simulink model "DEMOSYSTEM"  (R2015b)
settings: Solver=ode3  StartTime=0.0  StopTime=inf  FixedStep=T  RelTol=1e-3
InitFcn:
  | clear variables
  | T = 0.005; %Sampling time
  | 
  | % Impact detect subsys
  | %footExtensionRange = 17;        % 17[deg] hip angle at which foot extends/retracts
  | impactGeometryCondition = 10;   % 10 [deg] angle for geometric condition to check for impacts
  | impactGeometryConditionTol = 1; % 1 [deg] tolerance for impactGeometryCondition
  | 
  | impactCondi1 = 9*pi/180; % 9 [rad] retract
  | impactCondi2 = 1*pi/180; % 1 [rad] extend
  | 
  | % VC subsys
  | st_range = pi/18;
  | theta_retract = st_range;
  | theta_extend = -1*pi/180;
  | 
  | %refGenCoeffs = [ -1.0000, -0.9000, -1.0000, -1.2000, 1.9000, 2.4000, 1.3000, 1.1000, 1.0000];% MSC
  | refGenCoeffs = [ -1.0000, -0.9659, -0.8000, -0.8000, 1.3000, 1.4000, 1.3000, 1.2000, 1.0000];% Justin - slow
  | 
  | % PID subsys
  | feedbackP = 0.3;
  | feedbackD = 0.092;
  | 
  | % Observer gains
  | L1 = 200;
  | L2 = 10000;
  | A = [ 0 1 ;  0 0 ];
  | C = [ 1 0 ];
StopFcn:
  | % save file to results folder if it ran for longer than 10 seconds
  | 
  | %if(controlData.ref.Time(end) > 10)
  | %  name = datestr(now);
  | %  name = strrep(name,' ','_');
  | %  name = strrep(name,':','-');
  | %  name = strcat('results/',name);
  | %  save(name)
  | %end
  | 
  | %% display demo mode params:
  | disp('=====DEMO MODE=====');
undefined symbols (not defined in the file or in its folder): National_Instruments, PCI
libraries: simulink x8, sldrtlib x6, simulink_extras x1
settings Model: Creator=mounir  LastModifiedBy=mounir
settings DataIOCC: SaveFormat=Array
settings HardwareCC: ProdBitPerPointer=32  ProdLargestAtomicFloat=None  ProdIntDivRoundTo=Undefined  ProdEndianess=Unspecified  ProdWordSize=32  ProdHWDeviceType=32-bit Generic
settings GRTTargetCC: GeneratePreprocessorConditionals=Disable all
settings ConfigComp: CovModelRefEnable=Off

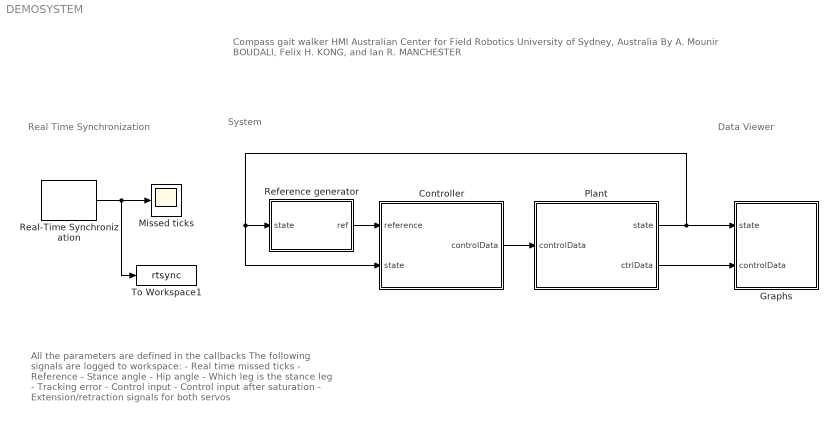
== system DEMOSYSTEM ==
  note: Compass gait walker HMI
      | Australian Center for Field Robotics
      | University of Sydney, Australia
      | By A. Mounir BOUDALI, Felix H. KONG, and Ian R. MANCHESTER
  note: All the parameters are defined in the callbacks
      |
      | The following signals are logged to workspace:
      | - Real time missed ticks
      | - Reference
      | - Stance angle
      | - Hip angle
      | - Which leg is the stance leg
      | - Tracking error
      | - Control input
      | - Control input after saturation
      | - Extension/retraction signals for both servos
  note: System
  note: Data Viewer
  note: Real Time Synchronization
  Controller : Subsystem
  Graphs : Subsystem
  Missed ticks : Scope
  Plant : Subsystem
  Real-Time Synchronization : sldrtlib/Real-Time Synchronization  SampleTime=T  MaxMissedTicks=100  ShowMissedTicks=on  YieldWhenWaiting=on
  Reference generator : Subsystem
  To Workspace1 : ToWorkspace  VariableName=rtsync  SaveFormat=Timeseries  SampleTime=T
  wires:
  Plant/1(state) -> Graphs/1(state), Reference generator/1(state), Controller/2(state)
  Controller/1(controlData) -> Plant/1(controlData)
  Reference generator/1(ref) -> Controller/1(reference)
  Real-Time Synchronization/1 -> Missed ticks/1, To Workspace1/1
  Plant/2(ctrlData) -> Graphs/2(controlData)

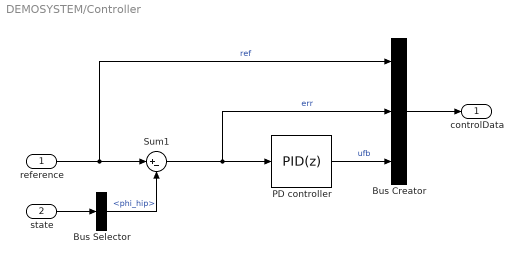
== system DEMOSYSTEM/Controller ==
  reference : Inport
  state : Inport  Port=2
  Bus Creator : BusCreator  Inputs=3
  Bus Selector : BusSelector  OutputSignals=phi_hip
  PD controller : simulink/Continuous/PID Controller  Controller=PID  TimeDomain=Discrete-time  SampleTime=T  IntegratorMethod=Forward Euler  FilterMethod=Forward Euler  Form=Ideal  UseFilter=on  ControllerParametersSource=internal  P=feedbackP  I=0  D=feedbackD  N=20  InitialConditionSource=internal  InitialConditionForIntegrator=0  InitialConditionForFilter=0  ExternalReset=none  LimitOutput=off  UpperSaturationLimit=inf  LowerSaturationLimit=-inf  LinearizeAsGain=on  AntiWindupMode=none  Kb=1  TrackingMode=off  Kt=1  PParamMin=[]  PParamMax=[]  IParamMin=[]  IParamMax=[]  DParamMin=[]  DParamMax=[]  NParamMin=[]  NParamMax=[]  KbParamMin=[]  KbParamMax=[]  KtParamMin=[]  KtParamMax=[]  POutMin=[]  POutMax=[]  IOutMin=[]  IOutMax=[]  DOutMin=[]  DOutMax=[]  NOutMin=[]  NOutMax=[]  KbOutMin=[]  KbOutMax=[]  KtOutMin=[]  KtOutMax=[]  IntegratorOutMin=[]  IntegratorOutMax=[]  FilterOutMin=[]  FilterOutMax=[]  SumOutMin=[]  SumOutMax=[]  SumI1OutMin=[]  SumI1OutMax=[]  SumI2OutMin=[]  SumI2OutMax=[]  SumI3OutMin=[]  SumI3OutMax=[]  SumDOutMin=[]  SumDOutMax=[]  SaturationOutMin=[]  SaturationOutMax=[]  IntegratorContinuousStateAttributes=''  IntegratorStateMustResolveToSignalObject=off  IntegratorRTWStateStorageClass=Auto  FilterContinuousStateAttributes=''  FilterStateMustResolveToSignalObject=off  FilterRTWStateStorageClass=Auto  DifferentiatorICPrevScaledInput=0  DifferentiatorOutMin=[]  DifferentiatorOutMax=[]
  Sum1 : Sum  Inputs=|+-
  controlData : Outport
  wires:
  state/1 -> Bus Selector/1
  Sum1/1 -> PD controller/1, Bus Creator/2  "err"
  reference/1 -> Sum1/1, Bus Creator/1  "ref"
  Bus Selector/1 -> Sum1/2  "<phi_hip>"
  Bus Creator/1 -> controlData/1
  PD controller/1 -> Bus Creator/3  "ufb"

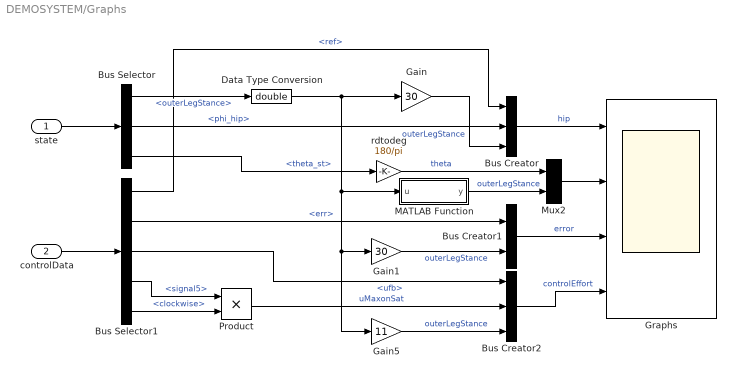
== system DEMOSYSTEM/Graphs ==
  state : Inport
  controlData : Inport  Port=2
  Bus Creator : BusCreator  Inputs=3
  Bus Creator1 : BusCreator  Inputs=2
  Bus Creator2 : BusCreator  Inputs=3
  Bus Selector : BusSelector  OutputSignals=outerLegStance,phi_hip,theta_st
  Bus Selector1 : BusSelector  OutputSignals=ref,err,ufb,signal5,clockwise
  Data Type Conversion : DataTypeConversion  OutDataTypeStr=double
  Gain : Gain  Gain=30
  Gain1 : Gain  Gain=30
  Gain5 : Gain  Gain=11
  Graphs : Scope  NumInputPorts=4
  MATLAB Function : MATLAB Function  TreatAsAtomicUnit=on
  Mux2 : Mux  Inputs=2
  Product : Product
  rdtodeg : Gain  Gain=180/pi
  wires:
  Bus Selector1/4 -> Product/1  "<signal5>"
  state/1 -> Bus Selector/1
  Bus Selector1/1 -> Bus Creator/1  "<ref>"
  Bus Selector/3 -> rdtodeg/1  "<theta_st>"
  Data Type Conversion/1 -> Gain5/1, Gain1/1, MATLAB Function/1(u), Gain/1
  Bus Selector/1 -> Data Type Conversion/1  "<outerLegStance>"
  Bus Selector/2 -> Bus Creator/2  "<phi_hip>"
  Bus Selector1/3 -> Bus Creator2/1  "<ufb>"
  controlData/1 -> Bus Selector1/1
  Bus Creator/1 -> Graphs/1  "hip"
  Gain/1 -> Bus Creator/3  "outerLegStance"
  Bus Creator1/1 -> Graphs/3  "error"
  Bus Selector1/2 -> Bus Creator1/1  "<err>"
  Gain1/1 -> Bus Creator1/2  "outerLegStance"
  Bus Creator2/1 -> Graphs/4  "controlEffort"
  Bus Selector1/5 -> Product/2  "<clockwise>"
  Product/1 -> Bus Creator2/2  "uMaxonSat"
  rdtodeg/1 -> Mux2/1  "theta"
  Gain5/1 -> Bus Creator2/3  "outerLegStance"
  Mux2/1 -> Graphs/2
  MATLAB Function/1(y) -> Mux2/2  "outerLegStance"

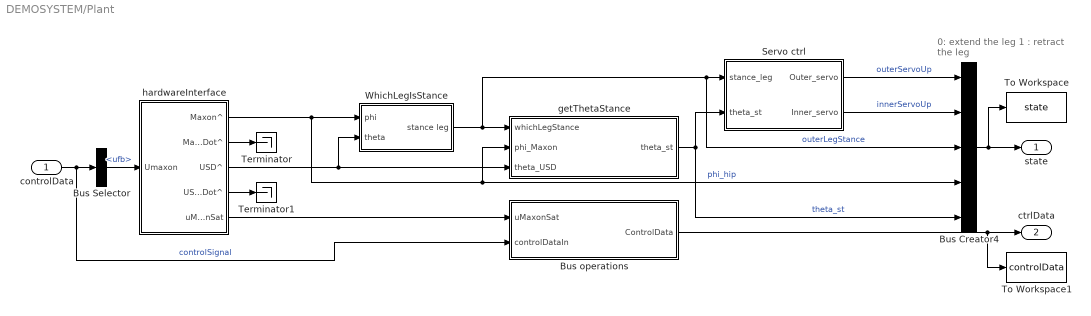
== system DEMOSYSTEM/Plant ==
  note: 0: extend the leg
      | 1 : retract the leg
  controlData : Inport
  Bus Creator4 : BusCreator  Inputs=5
  Bus Selector : BusSelector  OutputSignals=ufb
  Bus operations : Subsystem
  Servo ctrl : Subsystem
  Terminator : Terminator
  Terminator1 : Terminator
  To Workspace : ToWorkspace  VariableName=state  SaveFormat=Timeseries  SampleTime=T
  To Workspace1 : ToWorkspace  VariableName=controlData  SaveFormat=Timeseries  SampleTime=T
  WhichLegIsStance : Subsystem
  getThetaStance : Subsystem
  hardwareInterface : Subsystem
  state : Outport
  ctrlData : Outport  Port=2
  wires:
  hardwareInterface/1(Maxon^) -> getThetaStance/2(phi_Maxon), Bus Creator4/4, WhichLegIsStance/1(phi)  "phi_hip"
  WhichLegIsStance/1(stance leg) -> Bus Creator4/3, Servo ctrl/1(stance_leg), getThetaStance/1(whichLegStance)  "outerLegStance"
  getThetaStance/1(theta_st) -> Servo ctrl/2(theta_st), Bus Creator4/5  "theta_st"
  Bus Selector/1 -> hardwareInterface/1(Umaxon)  "<ufb>"
  hardwareInterface/3(USD^) -> WhichLegIsStance/2(theta), getThetaStance/3(theta_USD)
  controlData/1 -> Bus operations/2(controlDataIn), Bus Selector/1  "controlSignal"
  Bus Creator4/1 -> state/1, To Workspace/1
  Servo ctrl/1(Outer_servo) -> Bus Creator4/1  "outerServoUp"
  Servo ctrl/2(Inner_servo) -> Bus Creator4/2  "innerServoUp"
  Bus operations/1(ControlData) -> ctrlData/1, To Workspace1/1
  hardwareInterface/5(uMaxonSat) -> Bus operations/1(uMaxonSat)
  hardwareInterface/2(MaxonDot^) -> Terminator/1
  hardwareInterface/4(USDDot^) -> Terminator1/1

== system DEMOSYSTEM/Reference generator ==
  state : Inport
  Bezier Evaluation n Control Points : MATLAB Function  TreatAsAtomicUnit=on  SystemSampleTime=T
  Bus Selector : BusSelector  OutputSignals=outerLegStance,theta_st
  referencePostProc : Subsystem
  ref : Outport
  wires:
  Bus Selector/2 -> Bezier Evaluation n Control Points/1(idxAngle)  "<theta_st>"
  state/1 -> Bus Selector/1
  Bus Selector/1 -> referencePostProc/1(outerLegStance)  "<outerLegStance>"
  referencePostProc/1(refOut) -> ref/1
  Bezier Evaluation n Control Points/1(y) -> referencePostProc/2(refIn)  "ref out"

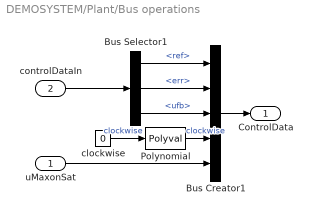
== system DEMOSYSTEM/Plant/Bus operations ==
  uMaxonSat : Inport
  controlDataIn : Inport  Port=2
  Bus Creator1 : BusCreator  Inputs='ref','err','ufb','clockwise','uMaxonSat'
  Bus Selector1 : BusSelector  OutputSignals=ref,err,ufb
  Polynomial : Polyval  Coefs=[2 -1]
  clockwise : Constant  Value=0
  ControlData : Outport
  wires:
  uMaxonSat/1 -> Bus Creator1/5
  Bus Creator1/1 -> ControlData/1
  Bus Selector1/1 -> Bus Creator1/1  "<ref>"
  Bus Selector1/3 -> Bus Creator1/3  "<ufb>"
  Bus Selector1/2 -> Bus Creator1/2  "<err>"
  controlDataIn/1 -> Bus Selector1/1
  clockwise/1 -> Polynomial/1  "clockwise"
  Polynomial/1 -> Bus Creator1/4  "clockwise"

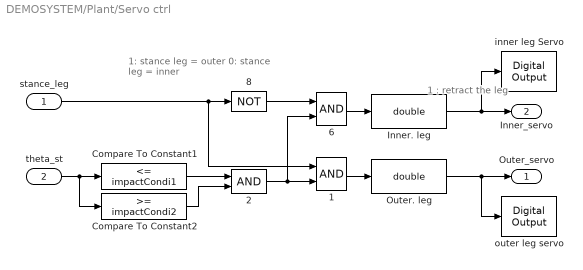
== system DEMOSYSTEM/Plant/Servo ctrl ==
  note: 1 : retract the leg
  note: 1: stance leg = outer
      | 0: stance leg = inner
  stance_leg : Inport
  theta_st : Inport  Port=2
  1 : Logic  AllPortsSameDT=off  OutDataTypeStr=boolean
  2 : Logic  AllPortsSameDT=off  OutDataTypeStr=boolean
  6 : Logic  AllPortsSameDT=off  OutDataTypeStr=boolean
  8 : Logic  Operator=NOT  Inputs=3  AllPortsSameDT=off  OutDataTypeStr=boolean
  Compare To Constant1 : simulink/Logic and Bit Operations/Compare To Constant  relop=<=  const=impactCondi1  OutDataTypeStr=boolean
  Compare To Constant2 : simulink/Logic and Bit Operations/Compare To Constant  relop=>=  const=impactCondi2  OutDataTypeStr=boolean
  Inner. leg : DataTypeConversion  OutDataTypeStr=double
  Outer. leg : DataTypeConversion  OutDataTypeStr=double
  inner leg Servo : sldrtlib/Digital Output  SampleTime=T  MaxMissedTicks=Inf  ShowMissedTicks=off  YieldWhenWaiting=on  DrvName=National_Instruments/PCI-6221  DrvAddress=4294967295  DrvOptions=[0 51 0 2 2]  Channels=1  BitMode=1  InitialValue=0  FinalValue=0
      settings: AttributesFormatString=National Instruments\nPCI-6221 [auto]
  outer leg servo : sldrtlib/Digital Output  SampleTime=T  MaxMissedTicks=Inf  ShowMissedTicks=off  YieldWhenWaiting=on  DrvName=National_Instruments/PCI-6221  DrvAddress=4294967295  DrvOptions=[0 51 0 2 2]  Channels=5  BitMode=1  InitialValue=0  FinalValue=0
      settings: AttributesFormatString=National Instruments\nPCI-6221 [auto]
  Outer_servo : Outport
  Inner_servo : Outport  Port=2
  wires:
  6/1 -> Inner. leg/1
  1/1 -> Outer. leg/1
  stance_leg/1 -> 8/1, 1/1
  8/1 -> 6/1
  2/1 -> 6/2, 1/2
  Compare To Constant1/1 -> 2/1
  Compare To Constant2/1 -> 2/2
  theta_st/1 -> Compare To Constant2/1, Compare To Constant1/1
  Outer. leg/1 -> Outer_servo/1, outer leg servo/1
  Inner. leg/1 -> Inner_servo/1, inner leg Servo/1

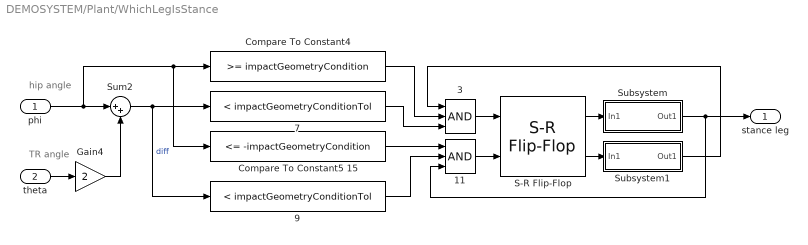
== system DEMOSYSTEM/Plant/WhichLegIsStance ==
  note: TR angle
  note: hip angle
  phi : Inport
  theta : Inport  Port=2
  11 : Logic  Inputs=3  AllPortsSameDT=off  OutDataTypeStr=boolean
  3 : Logic  Inputs=3  AllPortsSameDT=off  OutDataTypeStr=boolean
  7 : simulink/Logic and Bit Operations/Compare To Constant  relop=<  const=impactGeometryConditionTol  OutDataTypeStr=boolean
  9 : simulink/Logic and Bit Operations/Compare To Constant  relop=<  const=impactGeometryConditionTol  OutDataTypeStr=boolean
  Compare To Constant4 : simulink/Logic and Bit Operations/Compare To Constant  relop=>=  const=impactGeometryCondition  OutDataTypeStr=boolean
  Compare To Constant5 15 : simulink/Logic and Bit Operations/Compare To Constant  relop=<=  const=-impactGeometryCondition  OutDataTypeStr=boolean
  Gain4 : Gain  Gain=2
  S-R Flip-Flop : simulink_extras/Flip Flops/S-R Flip-Flop  initial_condition=0
  Subsystem : Subsystem
  Subsystem1 : Subsystem
  Sum2 : Sum  Inputs=|++
  stance leg : Outport
  wires:
  theta/1 -> Gain4/1
  Gain4/1 -> Sum2/2
  Compare To Constant4/1 -> 3/2
  S-R Flip-Flop/2 -> Subsystem1/1(In1)
  3/1 -> S-R Flip-Flop/1
  11/1 -> S-R Flip-Flop/2
  Compare To Constant5 15/1 -> 11/1
  9/1 -> 11/2
  7/1 -> 3/3
  S-R Flip-Flop/1 -> Subsystem/1(In1)
  Sum2/1 -> 7/1, 9/1  "diff"
  Subsystem/1(Out1) -> stance leg/1, 11/3
  Subsystem1/1(Out1) -> 3/1
  phi/1 -> Sum2/1, Compare To Constant5 15/1, Compare To Constant4/1

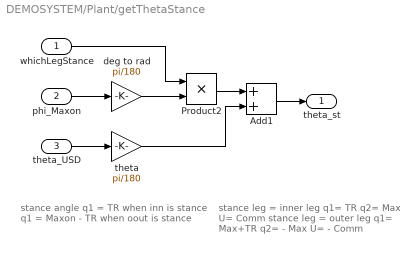
== system DEMOSYSTEM/Plant/getThetaStance ==
  note: stance leg = inner leg
      | q1= TR         q2= Max       U= Comm
      | stance leg = outer leg
      | q1= Max+TR  q2= - Max   U= - Comm
  note: stance angle
      | q1 = TR when inn is stance
      | q1 = Maxon - TR when oout is stance
  whichLegStance : Inport
  phi_Maxon : Inport  Port=2
  theta_USD : Inport  Port=3
  Add1 : Sum
  Product2 : Product  RndMeth=Zero
  deg to rad : Gain  Gain=pi/180
  theta : Gain  Gain=pi/180
  theta_st : Outport
  wires:
  Product2/1 -> Add1/1
  phi_Maxon/1 -> deg to rad/1
  theta_USD/1 -> theta/1
  whichLegStance/1 -> Product2/1
  theta/1 -> Add1/2
  deg to rad/1 -> Product2/2
  Add1/1 -> theta_st/1

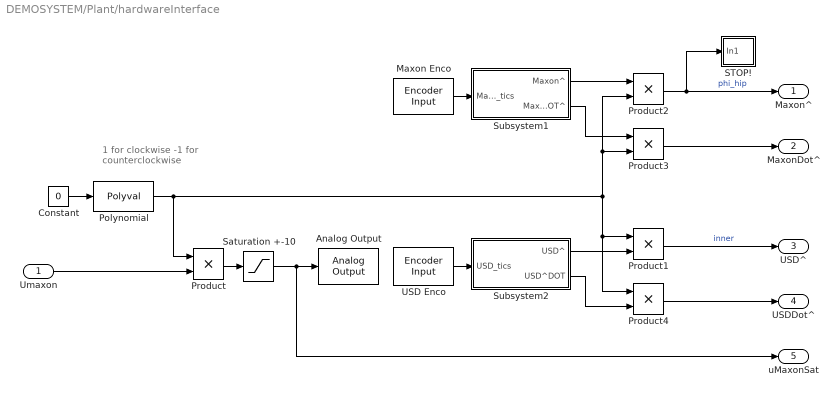
== system DEMOSYSTEM/Plant/hardwareInterface ==
  note: 1 for clockwise
      | -1 for counterclockwise
  Umaxon : Inport
  Analog Output : sldrtlib/Analog Output  SampleTime=T  MaxMissedTicks=Inf  ShowMissedTicks=off  YieldWhenWaiting=on  DrvName=National_Instruments/PCI-6221  DrvAddress=4294967295  DrvOptions=[0 51 0 2 2]  Channels=1  RangeMode=1  VoltRange=1  InitialValue=0  FinalValue=0
      settings: AttributesFormatString=National Instruments\nPCI-6221 [auto]
  Constant : Constant  Value=0
  Maxon Enco : sldrtlib/Encoder Input  SampleTime=T  MaxMissedTicks=Inf  ShowMissedTicks=off  YieldWhenWaiting=on  DrvName=National_Instruments/PCI-6221  DrvAddress=4294967295  DrvOptions=[0 51 0 2 2]  Channels=1  QuadMode=3  IndexPulse=2  InputFilter=Inf  DataType=1
      settings: AttributesFormatString=National Instruments\nPCI-6221 [auto]
  Polynomial : Polyval  Coefs=[2 -1]
  Product{,1..4} (5 alike) : Product  RndMeth=Zero
  STOP! : Subsystem
  Saturation +-10 : Saturate  UpperLimit=10  LowerLimit=-10
  Subsystem1 : Subsystem
  Subsystem2 : Subsystem
  USD Enco : sldrtlib/Encoder Input  SampleTime=T  MaxMissedTicks=Inf  ShowMissedTicks=off  YieldWhenWaiting=on  DrvName=National_Instruments/PCI-6221  DrvAddress=4294967295  DrvOptions=[0 51 0 2 2]  Channels=2  QuadMode=3  IndexPulse=2  InputFilter=Inf  DataType=1
      settings: AttributesFormatString=National Instruments\nPCI-6221 [auto]
  Maxon^ : Outport
  MaxonDot^ : Outport  Port=2
  USD^ : Outport  Port=3
  USDDot^ : Outport  Port=4
  uMaxonSat : Outport  Port=5
  wires:
  Constant/1 -> Polynomial/1
  Saturation +-10/1 -> uMaxonSat/1, Analog Output/1
  Umaxon/1 -> Product/2
  Maxon Enco/1 -> Subsystem1/1(Maxon_tics)
  USD Enco/1 -> Subsystem2/1(USD_tics)
  Subsystem2/1(USD^) -> Product1/2
  Subsystem1/1(Maxon^) -> Product2/1
  Polynomial/1 -> Product3/2, Product2/2, Product4/1, Product1/1, Product/1
  Product2/1 -> Maxon^/1, STOP!/1(In1)  "phi_hip"
  Product/1 -> Saturation +-10/1
  Product1/1 -> USD^/1  "inner"
  Product3/1 -> MaxonDot^/1
  Subsystem1/2(MaxonDOT^) -> Product3/1
  Product4/1 -> USDDot^/1
  Subsystem2/2(USD^DOT) -> Product4/2

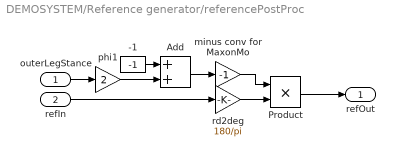
== system DEMOSYSTEM/Reference generator/referencePostProc ==
  outerLegStance : Inport  SampleTime=T
  refIn : Inport  Port=2  SampleTime=T
  -1 : Constant  Value=-1
  Add : Sum
  Product : Product  RndMeth=Zero
  minus conv for MaxonMo : Gain  Gain=-1
  phi1 : Gain  Gain=2
  rd2deg : Gain  Gain=180/pi
  refOut : Outport
  wires:
  refIn/1 -> rd2deg/1
  rd2deg/1 -> Product/2
  phi1/1 -> Add/2
  -1/1 -> Add/1
  Add/1 -> minus conv for MaxonMo/1
  outerLegStance/1 -> phi1/1
  minus conv for MaxonMo/1 -> Product/1
  Product/1 -> refOut/1

== system DEMOSYSTEM/Plant/WhichLegIsStance/Subsystem ==
  In1 : Inport
  Transport Delay : TransportDelay  DelayTime=T
  left leg3 : DataTypeConversion  OutDataTypeStr=double
  left leg4 : DataTypeConversion  OutDataTypeStr=boolean
  Out1 : Outport
  wires:
  Transport Delay/1 -> left leg4/1
  left leg3/1 -> Transport Delay/1
  In1/1 -> left leg3/1
  left leg4/1 -> Out1/1

== system DEMOSYSTEM/Plant/WhichLegIsStance/Subsystem1 ==
  In1 : Inport
  Transport Delay1 : TransportDelay  DelayTime=T
  left leg1 : DataTypeConversion  OutDataTypeStr=double
  left leg2 : DataTypeConversion  OutDataTypeStr=boolean
  Out1 : Outport
  wires:
  Transport Delay1/1 -> left leg2/1
  In1/1 -> left leg1/1
  left leg1/1 -> Transport Delay1/1
  left leg2/1 -> Out1/1

== system DEMOSYSTEM/Plant/hardwareInterface/STOP! ==
  note: Stop the experiment if the hip angle exceeds 120deg
  In1 : Inport
  " " : Stop
  120d : simulink/Logic and Bit Operations/Compare To Constant  relop=>=  const=120  OutDataTypeStr=boolean
  Abs : Abs
  wires:
  Abs/1 -> 120d/1
  120d/1 -> " "/1
  In1/1 -> Abs/1

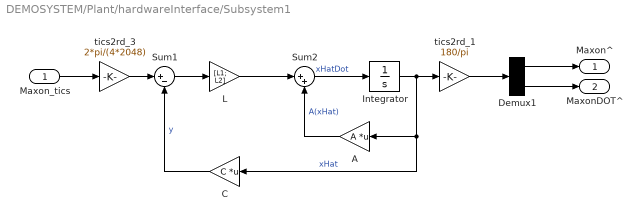
== system DEMOSYSTEM/Plant/hardwareInterface/Subsystem1 ==
  Maxon_tics : Inport
  A : Gain  Gain=A  Multiplication=Matrix(K*u)
  C : Gain  Gain=C  Multiplication=Matrix(K*u)
  Demux1 : Demux  Outputs=2
  Integrator : Integrator  InitialCondition=[0;0]
  L : Gain  Gain=[L1; L2]
  Sum1 : Sum  Inputs=|+-
  Sum2 : Sum  Inputs=|++
  tics2rd_1 : Gain  Gain=180/pi
  tics2rd_3 : Gain  Gain=2*pi/(4*2048)
  Maxon^ : Outport
  MaxonDOT^ : Outport  Port=2
  wires:
  Demux1/2 -> MaxonDOT^/1
  Demux1/1 -> Maxon^/1
  tics2rd_3/1 -> Sum1/1
  L/1 -> Sum2/1
  Sum2/1 -> Integrator/1  "xHatDot"
  Sum1/1 -> L/1
  C/1 -> Sum1/2  "y"
  Integrator/1 -> C/1, A/1, tics2rd_1/1  "xHat"
  A/1 -> Sum2/2  "A(xHat)"
  Maxon_tics/1 -> tics2rd_3/1
  tics2rd_1/1 -> Demux1/1

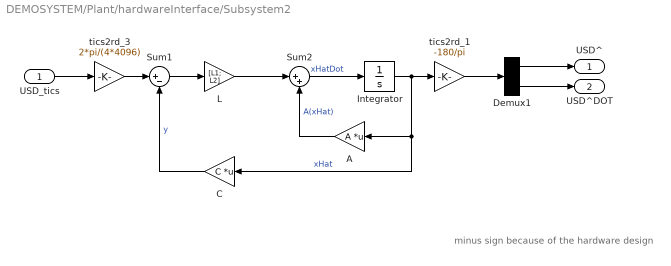
== system DEMOSYSTEM/Plant/hardwareInterface/Subsystem2 ==
  note: minus sign because of the hardware design
  USD_tics : Inport
  A : Gain  Gain=A  Multiplication=Matrix(K*u)
  C : Gain  Gain=C  Multiplication=Matrix(K*u)
  Demux1 : Demux  Outputs=2
  Integrator : Integrator  InitialCondition=[0;0]
  L : Gain  Gain=[L1; L2]
  Sum1 : Sum  Inputs=|+-
  Sum2 : Sum  Inputs=|++
  tics2rd_1 : Gain  Gain=-180/pi
  tics2rd_3 : Gain  Gain=2*pi/(4*4096)
  USD^ : Outport
  USD^DOT : Outport  Port=2
  wires:
  tics2rd_1/1 -> Demux1/1
  USD_tics/1 -> tics2rd_3/1
  A/1 -> Sum2/2  "A(xHat)"
  Integrator/1 -> tics2rd_1/1, A/1, C/1  "xHat"
  C/1 -> Sum1/2  "y"
  Sum1/1 -> L/1
  Sum2/1 -> Integrator/1  "xHatDot"
  L/1 -> Sum2/1
  tics2rd_3/1 -> Sum1/1
  Demux1/1 -> USD^/1
  Demux1/2 -> USD^DOT/1

== matlab function DEMOSYSTEM/Graphs/MATLAB Function ==
  data: u input; y output
function y = fcn(u)
%#codegen

y = 40*(u-0.5);

== matlab function DEMOSYSTEM/Reference generator/Bezier Evaluation n Control Points ==
  data: refGenCoeffs parameter; st_range parameter; idxAngle input; y output
%% Reference generation block - Virtual Holonomic Constraint
% this block takes theta stance as a phase variable and gives the desired trajectory for the hip angle
function y  = fcn(refGenCoeffs, st_range, idxAngle)

%
% refGenCoeffs      [nx1] [deg] reference trajectory expressed as a bezier curve
% st_Range          [1x1] [rad] nominal stance ankle angle range
% idxAngle          [1x1] [rad] current index angle (i.e. st. ankle angle)

theta_min    = st_range; % [rad]
theta_max    = -st_range;
refGenCoeffs = reshape(refGenCoeffs, length(refGenCoeffs),1);% ensure refGenCoeffs is a column vector
A            = 2*theta_min*refGenCoeffs; % bezier control points 
C            = 0.0; 
n            = size(A,1)-1;

if idxAngle < theta_max % [rad] Saturate the phase if the step lenght is bigger than stance range
    s = 1;
 elseif idxAngle > theta_min
    s = 0;
 else
    s = (idxAngle-theta_min)/(theta_max-theta_min);% s--> [0:1]
end

for k = 0:n
  C = C+A(k+1)*s.^(k).*(1-s).^(n-k)*gamma(n+1)/(gamma(n-k+1)*gamma(k+1));% hip reference 
end

    y = C;
